simulink model "basic"  (R2018a)
settings: Solver=VariableStepAuto  StartTime=0.0  StopTime=200*ts  RelTol=1e-3  EnableMultiTasking=on
undefined symbols (not defined in the file): ts
libraries: simulink x1
settings Model: Creator=pablo  LastModifiedBy=pcoss
settings OptimizationCC: BlockReduction=off  ConditionallyExecuteInputs=off  DefaultParameterBehavior=Inlined  LifeSpan=inf
settings DebuggingCC: AlgebraicLoopMsg=error  SFUnexpectedBacktrackingDiag=warning  SFNoUnconditionalDefaultTransitionDiag=warning  SFExecutionAtInitializationDiag=none
settings HardwareCC: ProdBitPerPointer=32  ProdBitPerSizeT=32  ProdBitPerPtrDiffT=32  ProdLargestAtomicFloat=None  ProdIntDivRoundTo=Undefined  ProdEndianess=Unspecified  ProdWordSize=32  ProdHWDeviceType=ASIC/FPGA->ASIC/FPGA  ProdEqTarget=off
settings CodeAppCC: StateflowObjectComments=on
settings GRTTargetCC: TargetLangStandard=C89/C90 (ANSI)  GeneratePreprocessorConditionals=Disable all
settings ConfigComp: CovMetricSettings=dw  CovHtmlReporting=on  CovSaveCumulativeToWorkspaceVar=on  CovSaveSingleToWorkspaceVar=on  CovExternalEMLEnable=off

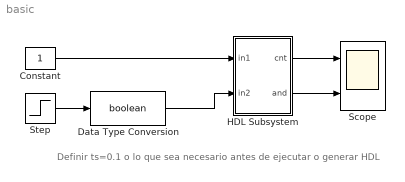
== system basic ==
  note: Definir ts=0.1 o lo que sea necesario antes de ejecutar o generar HDL
  Constant : Constant  OutDataTypeStr=boolean  SampleTime=ts
  Data Type Conversion : DataTypeConversion  OutDataTypeStr=boolean
  HDL Subsystem : Subsystem
  Scope : Scope  NumInputPorts=2
  Step : Step  Time=100*ts  SampleTime=ts
  wires:
  Constant/1 -> HDL Subsystem/1(in1)
  Step/1 -> Data Type Conversion/1
  HDL Subsystem/1(cnt) -> Scope/1
  HDL Subsystem/2(and) -> Scope/2
  Data Type Conversion/1 -> HDL Subsystem/2(in2)

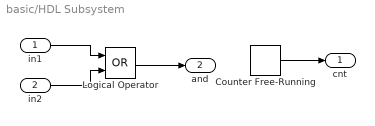
== system basic/HDL Subsystem ==
  in1 : Inport
  in2 : Inport  Port=2
  Counter Free-Running : simulink/Sources/Counter Free-Running  NumBits=4  tsamp=-1
  Logical Operator : Logic  Operator=OR  AllPortsSameDT=off  OutDataTypeStr=boolean
  cnt : Outport
  and : Outport  Port=2
  wires:
  Logical Operator/1 -> and/1
  in2/1 -> Logical Operator/2
  in1/1 -> Logical Operator/1
  Counter Free-Running/1 -> cnt/1
